simulink model "All_5converters"  (Simulink 7.9)
settings: Solver=ode45  StartTime=0.0  StopTime=1  RelTol=1e-3
libraries: powerlib x36
settings Model: Creator=spiro43  LastModifiedBy=spiro72
settings DebuggingCC: UnconnectedInputMsg=none  UnconnectedOutputMsg=none  UnconnectedLineMsg=none

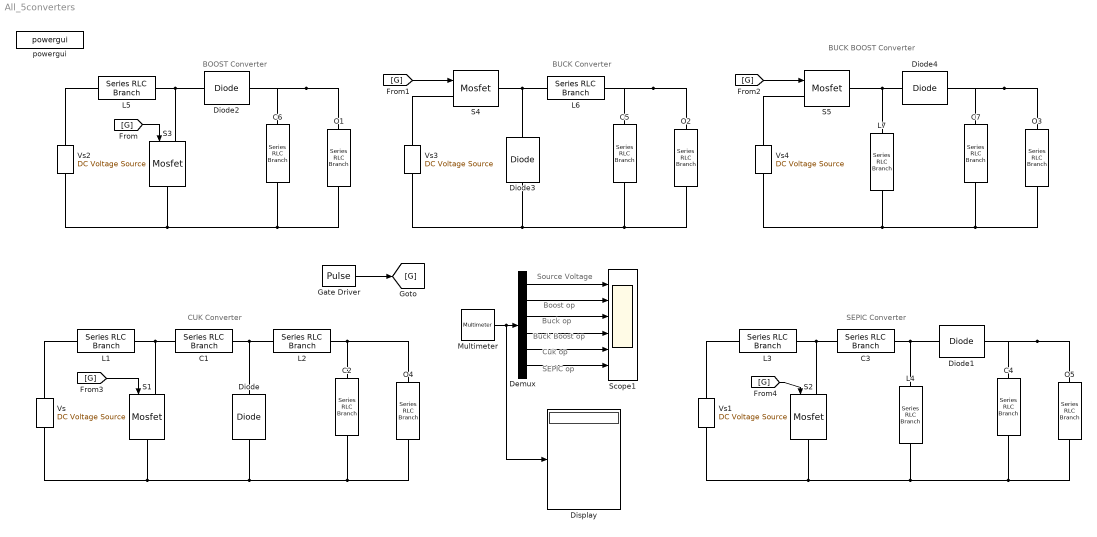
== system All_5converters ==
  note: CUK Converter
  note: SEPIC Converter
  note: BOOST Converter
  note: BUCK Converter
  note: BUCK BOOST Converter
  note: Source Voltage
  note: Boost op
  note: Buck op
  note: Buck Boost op
  note: Cuk op
  note: SEPIC op
  C1 : powerlib/Elements/Series RLC Branch  LConnTagsString=__new0  RConnTagsString=__new0  BranchType=C  Resistance=1  Inductance=1e-3  SetiL0=off  InitialCurrent=0  Capacitance=200e-6  Setx0=off  InitialVoltage=0  Measurements=None
  C{2,4..7} (5 alike) : powerlib/Elements/Series RLC Branch  LConnTagsString=__new0  RConnTagsString=__new0  BranchType=C  Resistance=1  Inductance=1e-3  SetiL0=off  InitialCurrent=0  Capacitance=220e-6  Setx0=off  InitialVoltage=0  Measurements=None
  C3 : powerlib/Elements/Series RLC Branch  LConnTagsString=__new0  RConnTagsString=__new0  BranchType=C  Resistance=1  Inductance=1e-3  SetiL0=off  InitialCurrent=0  Capacitance=200e-6  Setx0=off  InitialVoltage=0  Measurements=None
  Demux : Demux  Outputs=6
  Diode{,1..4} (5 alike) : powerlib/Power Electronics/Diode  Ron=0.001  Lon=0  Vf=0.8  IC=0  UseSnubber=off  Rs=500  Cs=250e-9  Measurements=off
  Display : Display
  Gate Driver : DiscretePulseGenerator  PulseType=Time based  Period=1/(25e3)  PulseWidth=40
  L{1..7} (7 alike) : powerlib/Elements/Series RLC Branch  LConnTagsString=__new0  RConnTagsString=__new0  BranchType=L  Resistance=1  Inductance=200e-6  SetiL0=off  InitialCurrent=0  Capacitance=1e-6  Setx0=off  InitialVoltage=0  Measurements=None
  Multimeter : powerlib/Measurements/Multimeter  PhasorSimulation=off  OutputType=Complex  sel=[10 1 2 3 4 5]  L=10  Gain=[1 1 1 1 1 1]  yselected={'Usrc: Vs','Ub: O1','Ub: O2','Ub: O3','Ub: O4','Ub: O5'};  PSBOutputType=1  PSBequivalent=0  AxesSetting=[0,0.1,-100,100]  Display=0  SavedBlockNames=-11
  O{1..5} (5 alike) : powerlib/Elements/Series RLC Branch  LConnTagsString=__new0  RConnTagsString=__new0  BranchType=R  Resistance=20  Inductance=1e-3  SetiL0=off  InitialCurrent=0  Capacitance=1e-6  Setx0=off  InitialVoltage=0  Measurements=Branch voltage
  S{1..5} (5 alike) : powerlib/Power Electronics/Mosfet  Ron=0.1  Lon=0  Rd=0.01  Vfd=0  IC=0  Rs=1e5  Cs=inf  Measurements=off
  Scope1 : Scope  NumInputPorts=6
      settings: YMin=22.3~-8.6~37.5~-5~-5~-5  YMax=23.9~-6.7~38.7~5~5~5
  Vs{,1..4} (5 alike) : powerlib/Electrical Sources/DC Voltage Source  Amplitude=20  Measurements=Voltage
  powergui : powerlib/powergui  SimulationMode=Continuous  SolverType=Tustin  SampleTime=50e-6  frequency=60  SPID=off  DisableSnubberDevices=off  DisableRonSwitches=off  DisableVfSwitches=off  SwTol=0  Interpol=off  DisplayEquations=off  FunctionMessages=off  frequencyindice=0  Pbase=100e6  ErrMax=1e-4  Iterations=50  UnitsV=kV  UnitsW=MW  echomessages=off  HookPort=off  EnableUseOfTLC=off  x0status=blocks  RestoreLinks=warning  ResistiveCurrentMeasurement=off  Frange=[0:2:500]  Ylog=off  Xlog=on  ShowGrid=off  save=off  variable=ZData  ZoomFFT=on  StartTime=0.0  cycles=1  DisplayStyle=1  fundamental=60  FreqAxis=off  MaxFrequency=1000  frequencyindicesteady=1  RmsSteady=1  display=off  Ts=0  methode=off
  wires:
  Multimeter/1 -> Demux/1, Display/1
  Demux/1 -> Scope1/1
  Demux/2 -> Scope1/2
  Demux/3 -> Scope1/3
  Demux/4 -> Scope1/4
  Demux/5 -> Scope1/5
  Demux/6 -> Scope1/6
  Gate Driver/1 -> [G]
  [G] -> S3/1
  [G] -> S4/1
  [G] -> S5/1
  [G] -> S1/1
  [G] -> S2/1
  connections:
  L1/RConn1 -- S1/LConn1 -- C1/LConn1
  Diode/RConn1 -- Vs/LConn1 -- S1/RConn1 -- O4/RConn1 -- C2/RConn1
  Diode/LConn1 -- L2/LConn1 -- C1/RConn1
  O4/LConn1 -- L2/RConn1 -- C2/LConn1
  L1/LConn1 -- Vs/RConn1
  C3/LConn1 -- L3/RConn1 -- S2/LConn1
  Vs1/LConn1 -- S2/RConn1 -- O5/RConn1 -- C4/RConn1 -- L4/RConn1
  L4/LConn1 -- C3/RConn1 -- Diode1/LConn1
  Diode1/RConn1 -- C4/LConn1 -- O5/LConn1
  Vs1/RConn1 -- L3/LConn1
  Diode2/LConn1 -- L5/RConn1 -- S3/LConn1
  O1/RConn1 -- C6/RConn1 -- Vs2/LConn1 -- S3/RConn1
  Diode2/RConn1 -- C6/LConn1 -- O1/LConn1
  L5/LConn1 -- Vs2/RConn1
  S4/RConn1 -- Diode3/RConn1 -- L6/LConn1
  O2/RConn1 -- C5/RConn1 -- Vs3/LConn1 -- Diode3/LConn1
  L6/RConn1 -- C5/LConn1 -- O2/LConn1
  S4/LConn1 -- Vs3/RConn1
  L7/LConn1 -- S5/RConn1 -- Diode4/RConn1
  L7/RConn1 -- O3/RConn1 -- C7/RConn1 -- Vs4/LConn1
  Diode4/LConn1 -- C7/LConn1 -- O3/LConn1
  S5/LConn1 -- Vs4/RConn1
